simulink model "Simulink_System5"  (R2020a)
settings: Solver=VariableStepAuto  StartTime=0.0  StopTime=800  MaxStep=0.1  RelTol=1e-3
undefined symbols (not defined in the file): kcA5, kcA6, kcA7, kcA8, kdA5, kdA6, kdA7, kdA8, kiA5, kiA6, kiA7, kiA8, Qin_1, Qin_2
libraries: cstblocks x4
settings Model: Creator=beto1  LastModifiedBy=beto1

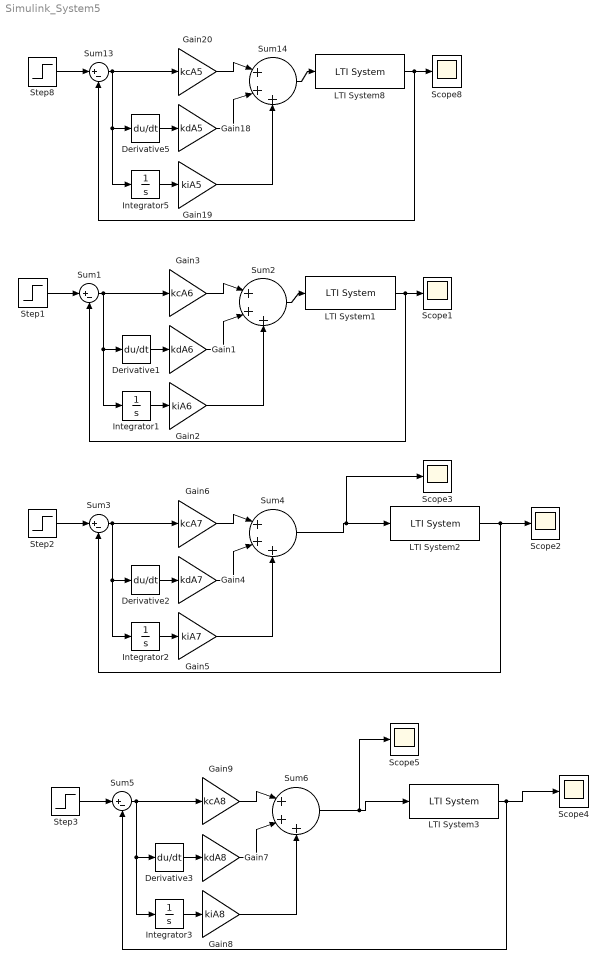
== system Simulink_System5 ==
  Derivative{1..3,5} (4 alike) : Derivative
  Gain1 : Gain  Gain=kdA6
  Gain18 : Gain  Gain=kdA5
  Gain19 : Gain  Gain=kiA5
  Gain2 : Gain  Gain=kiA6
  Gain20 : Gain  Gain=kcA5
  Gain3 : Gain  Gain=kcA6
  Gain4 : Gain  Gain=kdA7
  Gain5 : Gain  Gain=kiA7
  Gain6 : Gain  Gain=kcA7
  Gain7 : Gain  Gain=kdA8
  Gain8 : Gain  Gain=kiA8
  Gain9 : Gain  Gain=kcA8
  Integrator{1..3,5} (4 alike) : Integrator
  LTI System1 : cstblocks/LTI System  sys=H2  IC=[]
  LTI System2 : cstblocks/LTI System  sys=H1  IC=[]
  LTI System3 : cstblocks/LTI System  sys=H2  IC=[]
  LTI System8 : cstblocks/LTI System  sys=H1  IC=[]
  Scope{1..5,8} (6 alike) : Scope
  Step1 : Step  Time=0  After=Qin_2  SampleTime=0
  Step2 : Step  Time=0  After=Qin_1  SampleTime=0
  Step3 : Step  Time=0  After=Qin_2  SampleTime=0
  Step8 : Step  Time=0  After=Qin_1  SampleTime=0
  Sum{1,3,5,13} (4 alike) : Sum  Inputs=|+-
  Sum{2,4,6,14} (4 alike) : Sum  Inputs=|+++
  wires:
  Sum14/1 -> LTI System8/1
  Step8/1 -> Sum13/1
  LTI System8/1 -> Sum13/2, Scope8/1
  Derivative5/1 -> Gain18/1
  Integrator5/1 -> Gain19/1
  Gain18/1 -> Sum14/2
  Gain20/1 -> Sum14/1
  Gain19/1 -> Sum14/3
  Sum13/1 -> Integrator5/1, Derivative5/1, Gain20/1
  Sum1/1 -> Integrator1/1, Derivative1/1, Gain3/1
  Gain2/1 -> Sum2/3
  Integrator1/1 -> Gain2/1
  Gain3/1 -> Sum2/1
  Gain1/1 -> Sum2/2
  Step1/1 -> Sum1/1
  LTI System1/1 -> Sum1/2, Scope1/1
  Derivative1/1 -> Gain1/1
  Sum2/1 -> LTI System1/1
  Sum3/1 -> Integrator2/1, Derivative2/1, Gain6/1
  Gain5/1 -> Sum4/3
  Integrator2/1 -> Gain5/1
  Gain6/1 -> Sum4/1
  Gain4/1 -> Sum4/2
  Step2/1 -> Sum3/1
  LTI System2/1 -> Sum3/2, Scope2/1
  Derivative2/1 -> Gain4/1
  Sum4/1 -> Scope3/1, LTI System2/1
  Step3/1 -> Sum5/1
  Gain7/1 -> Sum6/2
  Sum6/1 -> Scope5/1, LTI System3/1
  Derivative3/1 -> Gain7/1
  LTI System3/1 -> Sum5/2, Scope4/1
  Sum5/1 -> Integrator3/1, Derivative3/1, Gain9/1
  Gain9/1 -> Sum6/1
  Gain8/1 -> Sum6/3
  Integrator3/1 -> Gain8/1
